simulink model "sampleModel2084"  (R2023a)
settings: Solver=VariableStepAuto  StartTime=0.0  StopTime=10.0  RelTol=1e-3
libraries: hdlsllib x5, simulink x3
settings Model: Creator=user1  LastModifiedBy=user1

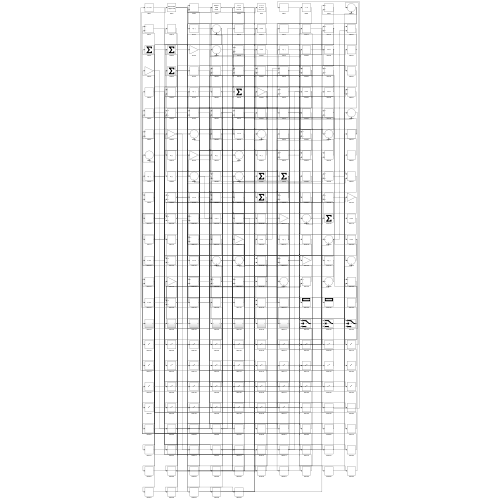
[thumbnail: Simulink's stored preview of the top-level diagram]
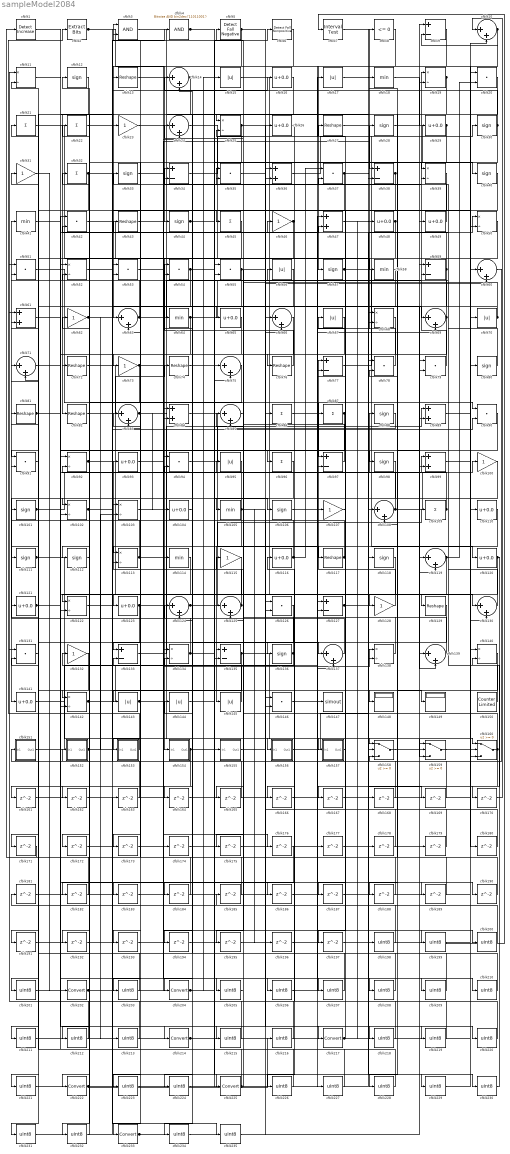
== system sampleModel2084 ==
  cfblk1 : simulink/Logic and Bit Operations/Detect Increase  vinit=0.0  OutDataTypeStr=boolean
      settings: LibrarySourceBlock=|
      | hdlsllib/Logic and Bit
      | Operations/Detect
      | Increase
  cfblk{10,14,24,60,63,66,69,71,75,83,85,108,119,124..125,130,137,139} (18 alike) : Sum  Inputs=|++
  cfblk{23,31,46,62,73,100,107,115,128,132} (10 alike) : Gain
  cfblk{12,28,30,33,40,44,57,80,88,98,101,106,111..112,118,136} (16 alike) : Signum
  cfblk{11,19,25,39,50,52,68,92,102..103,113,122,134,138,140,142} (16 alike) : Product  Inputs=*/  RndMeth=Zero  SaturateOnIntegerOverflow=on
  cfblk{16,26,29,48..49,65,93,104,110,116,120..121,123,141} (14 alike) : Bias  Bias=0.0  SaturateOnIntegerOverflow=off
  cfblk{18,41,58,64,105,114} (6 alike) : MinMax
  cfblk{21..22,32,45,86..87,96,109} (8 alike) : Sum  Inputs=+
  cfblk{13,27,43,72,74,76,81..82,117,129} (10 alike) : Reshape
  cfblk{20,35,37,42,51,53..55,78..79,90..91,94,126,131,146} (16 alike) : DotProduct  OutDataTypeStr=Inherit: Inherit via internal rule
  cfblk{9,34,38,59,77,97,127,133,135} (9 alike) : Sum  Inputs=+-
  cfblk{15,17,56,67,70,95,143..145} (9 alike) : Abs  SaturateOnIntegerOverflow=off
  cfblk147 : ToWorkspace  VariableName=simout  SaveFormat=Timeseries  SampleTime=-1
  cfblk148 : Display
  cfblk149 : Display
  cfblk150 : hdlsllib/Sources/Counter Limited  uplimit=7  tsamp=-1
  cfblk151 : Subsystem
      settings: LibrarySourceBlock=|
      | hdlsllib/Ports &
      | Subsystems/Subsystem
  cfblk152 : Subsystem
      settings: LibrarySourceBlock=|
      | hdlsllib/Ports &
      | Subsystems/Subsystem
  cfblk153 : Subsystem
      settings: LibrarySourceBlock=|
      | hdlsllib/Ports &
      | Subsystems/Subsystem
  cfblk154 : Subsystem
      settings: LibrarySourceBlock=|
      | hdlsllib/Ports &
      | Subsystems/Subsystem
  cfblk155 : Subsystem
      settings: LibrarySourceBlock=|
      | hdlsllib/Ports &
      | Subsystems/Subsystem
  cfblk156 : Subsystem
      settings: LibrarySourceBlock=|
      | hdlsllib/Ports &
      | Subsystems/Subsystem
  cfblk157 : Subsystem
      settings: LibrarySourceBlock=|
      | hdlsllib/Ports &
      | Subsystems/Subsystem
  cfblk158 : Switch  SaturateOnIntegerOverflow=off  InputSameDT=off
  cfblk159 : Switch  SaturateOnIntegerOverflow=off  InputSameDT=off
  cfblk160 : Switch  SaturateOnIntegerOverflow=off  InputSameDT=off
  cfblk{161..197} (37 alike) : Delay  SampleTime=1
  cfblk{198..201,203,205..213,215..216,218..221,223..224,226..232,234..235} (31 alike) : DataTypeConversion  OutDataTypeStr=uint8  SaturateOnIntegerOverflow=off  RndMeth=Floor
  cfblk2 : simulink/Logic and Bit Operations/Extract Bits  bitsToExtract=Upper half  numBits=8  bitIdxRange=[0 7]  outScalingMode=Preserve fixed-point scaling
      settings: LibrarySourceBlock=|
      | hdlsllib/Logic and Bit
      | Operations/Extract Bits
  cfblk{202,204,214,217,222,225,233} (7 alike) : DataTypeConversion  SaturateOnIntegerOverflow=off  RndMeth=Floor
  cfblk3 : Logic  AllPortsSameDT=off  OutDataTypeStr=boolean
  cfblk{36,47,61,84,89,99} (6 alike) : Sum
  cfblk4 : simulink/Logic and Bit Operations/Bitwise Operator  logicop=AND  UseBitMask=on  BitMask=bin2dec('11011001')  BitMaskRealWorld=Stored Integer
      settings: LibrarySourceBlock=|
      | hdlsllib/Logic and Bit
      | Operations/Bitwise
      | Operator
  cfblk5 : hdlsllib/Logic and Bit Operations/Detect Fall Negative  vinit=0  OutDataTypeStr=boolean
  cfblk6 : hdlsllib/Logic and Bit Operations/Detect Fall Nonpositive  vinit=0  OutDataTypeStr=boolean
  cfblk7 : hdlsllib/Logic and Bit Operations/Interval Test  IntervalClosedRight=on  uplimit=0.5  IntervalClosedLeft=on  lowlimit=-0.5  OutDataTypeStr=boolean
  cfblk8 : hdlsllib/Logic and Bit Operations/Compare To Zero  relop=<=  OutDataTypeStr=boolean
  wires:
  cfblk20/1 -> cfblk82/1
  cfblk78/1 -> cfblk8/1
  cfblk100/1 -> cfblk141/1
  cfblk153/1(Out1) -> cfblk2/1
  cfblk8/1 -> cfblk63/1
  cfblk60/1 -> cfblk151/1(In1)
  cfblk117/1 -> cfblk41/1, cfblk64/1
  cfblk130/1 -> cfblk33/1
  cfblk5/1 -> cfblk13/1, cfblk38/2, cfblk98/1
  cfblk29/1 -> cfblk153/1(In1), cfblk76/1
  cfblk115/1 -> cfblk204/1
  cfblk79/1 -> cfblk19/1
  cfblk81/1 -> cfblk128/1, cfblk96/1
  cfblk13/1 -> cfblk156/1(In1)
  cfblk128/1 -> cfblk77/1
  cfblk25/1 -> cfblk130/1, cfblk122/1
  cfblk6/1 -> cfblk44/1
  cfblk72/1 -> cfblk129/1
  cfblk108/1 -> cfblk100/1, cfblk32/1
  cfblk73/1 -> cfblk28/1, cfblk90/1, cfblk172/1
  cfblk158/1 -> cfblk119/1
  cfblk77/1 -> cfblk30/1
  cfblk69/1 -> cfblk54/2, cfblk226/1
  cfblk9/1 -> cfblk57/1
  cfblk107/1 -> cfblk27/1
  cfblk21/1 -> cfblk154/1(In1)
  cfblk83/1 -> cfblk148/1, cfblk104/1
  cfblk52/1 -> cfblk225/1
  cfblk121/1 -> cfblk81/1, cfblk215/1
  cfblk56/1 -> cfblk123/1
  cfblk136/1 -> cfblk24/1, cfblk134/2
  cfblk127/1 -> cfblk50/1, cfblk159/3
  cfblk19/1 -> cfblk25/1, cfblk108/2
  cfblk64/1 -> cfblk56/1, cfblk142/2
  cfblk59/1 -> cfblk84/1, cfblk22/1
  cfblk84/1 -> cfblk117/1
  cfblk57/1 -> cfblk120/1, cfblk139/2
  cfblk24/1 -> cfblk147/1
  cfblk37/1 -> cfblk122/2, cfblk169/1
  cfblk68/1 -> cfblk133/1
  cfblk51/1 -> cfblk97/1
  cfblk109/1 -> cfblk62/1, cfblk18/1
  cfblk104/1 -> cfblk34/1
  cfblk36/1 -> cfblk9/1
  cfblk54/1 -> cfblk91/1, cfblk106/1, cfblk186/1
  cfblk10/1 -> cfblk127/2, cfblk160/2, cfblk9/2
  cfblk61/1 -> cfblk217/1
  cfblk34/1 -> cfblk17/1
  cfblk113/1 -> cfblk93/1, cfblk208/1
  cfblk14/1 -> cfblk72/1, cfblk221/1
  cfblk135/1 -> cfblk158/1, cfblk142/1
  cfblk15/1 -> cfblk107/1
  cfblk92/1 -> cfblk137/1, cfblk90/2
  cfblk82/1 -> cfblk74/1
  cfblk133/1 -> cfblk89/1
  cfblk1/1 -> cfblk23/1
  cfblk125/1 -> cfblk103/1, cfblk113/2
  cfblk105/1 -> cfblk102/1, cfblk113/1, cfblk196/1, cfblk207/1
  cfblk139/1 -> cfblk5/1
  cfblk156/1(Out1) -> cfblk78/1
  cfblk154/1(Out1) -> cfblk15/1, cfblk171/1
  cfblk48/1 -> cfblk94/1, cfblk101/1
  cfblk138/1 -> cfblk85/1
  cfblk120/1 -> cfblk143/1, cfblk170/1
  cfblk80/1 -> cfblk51/2
  cfblk2/1 -> cfblk24/2, cfblk99/2, cfblk50/2
  cfblk103/1 -> cfblk88/1
  cfblk97/1 -> cfblk3/1
  cfblk134/1 -> cfblk91/2, cfblk14/2, cfblk230/1
  cfblk76/1 -> cfblk54/1
  cfblk146/1 -> cfblk138/1
  cfblk30/1 -> cfblk39/1, cfblk14/1
  cfblk111/1 -> cfblk160/1, cfblk43/1
  cfblk110/1 -> cfblk145/1
  cfblk75/1 -> cfblk222/1
  cfblk43/1 -> cfblk149/1
  cfblk4/1 -> cfblk40/1, cfblk58/1
  cfblk32/1 -> cfblk16/1, cfblk146/2, cfblk111/1
  cfblk66/1 -> cfblk233/1
  cfblk28/1 -> cfblk110/1
  cfblk159/1 -> cfblk80/1
  cfblk31/1 -> cfblk202/1
  cfblk3/1 -> cfblk118/1
  cfblk143/1 -> cfblk138/2, cfblk39/2
  cfblk94/1 -> cfblk36/2
  cfblk119/1 -> cfblk20/2, cfblk125/2, cfblk232/1
  cfblk50/1 -> cfblk112/1
  cfblk27/1 -> cfblk38/1
  cfblk152/1(Out1) -> cfblk4/1, cfblk103/2, cfblk182/1
  cfblk102/1 -> cfblk12/1, cfblk205/1
  cfblk55/1 -> cfblk60/2, cfblk105/1, cfblk164/1
  cfblk42/1 -> cfblk108/1
  cfblk116/1 -> cfblk83/1, cfblk37/1
  cfblk89/1 -> cfblk10/2
  cfblk137/1 -> cfblk124/1
  cfblk87/1 -> cfblk102/2, cfblk173/1
  cfblk11/1 -> cfblk214/1
  cfblk155/1(Out1) -> cfblk126/1
  cfblk88/1 -> cfblk85/2
  cfblk95/1 -> cfblk124/2
  cfblk141/1 -> cfblk68/2
  cfblk38/1 -> cfblk34/2, cfblk45/1
  cfblk124/1 -> cfblk109/1, cfblk157/1(In1)
  cfblk142/1 -> cfblk69/2, cfblk192/1
  cfblk70/1 -> cfblk35/1, cfblk65/1
  cfblk33/1 -> cfblk134/1
  cfblk145/1 -> cfblk92/2
  cfblk160/1 -> cfblk95/1, cfblk197/1
  cfblk63/1 -> cfblk21/1, cfblk59/2
  cfblk151/1(Out1) -> cfblk53/2
  cfblk45/1 -> cfblk73/1
  cfblk46/1 -> cfblk136/1, cfblk83/2
  cfblk150/1 -> cfblk46/1
  cfblk123/1 -> cfblk190/1, cfblk191/1
  cfblk35/1 -> cfblk87/1
  cfblk118/1 -> cfblk135/1
  cfblk122/1 -> cfblk47/2
  cfblk18/1 -> cfblk29/1
  cfblk22/1 -> cfblk69/1
  cfblk101/1 -> cfblk49/1, cfblk99/1
  cfblk62/1 -> cfblk213/1, cfblk235/1
  cfblk49/1 -> cfblk35/2
  cfblk74/1 -> cfblk6/1
  cfblk44/1 -> cfblk114/1, cfblk160/3
  cfblk91/1 -> cfblk161/1
  cfblk161/1 -> cfblk130/2
  cfblk112/1 -> cfblk162/1
  cfblk162/1 -> cfblk89/2
  cfblk163/1 -> cfblk42/2
  cfblk164/1 -> cfblk19/2
  cfblk85/1 -> cfblk165/1
  cfblk165/1 -> cfblk53/1
  cfblk26/1 -> cfblk166/1
  cfblk166/1 -> cfblk127/1
  cfblk39/1 -> cfblk167/1
  cfblk167/1 -> cfblk159/2
  cfblk17/1 -> cfblk168/1
  cfblk168/1 -> cfblk68/1
  cfblk169/1 -> cfblk159/1
  cfblk170/1 -> cfblk10/1
  cfblk171/1 -> cfblk1/1
  cfblk172/1 -> cfblk139/1
  cfblk173/1 -> cfblk3/2
  cfblk126/1 -> cfblk175/1
  cfblk93/1 -> cfblk176/1
  cfblk177/1 -> cfblk79/2
  cfblk178/1 -> cfblk37/2
  cfblk179/1 -> cfblk78/2
  cfblk99/1 -> cfblk180/1
  cfblk180/1 -> cfblk36/1
  cfblk181/1 -> cfblk119/2
  cfblk182/1 -> cfblk92/1
  cfblk40/1 -> cfblk183/1
  cfblk183/1 -> cfblk20/1
  cfblk58/1 -> cfblk184/1
  cfblk184/1 -> cfblk133/2
  cfblk185/1 -> cfblk94/2
  cfblk186/1 -> cfblk137/2
  cfblk157/1(Out1) -> cfblk187/1
  cfblk187/1 -> cfblk77/2
  cfblk90/1 -> cfblk188/1
  cfblk188/1 -> cfblk63/2
  cfblk41/1 -> cfblk189/1
  cfblk189/1 -> cfblk51/1
  cfblk190/1 -> cfblk158/3
  cfblk191/1 -> cfblk135/2
  cfblk192/1 -> cfblk60/1
  cfblk67/1 -> cfblk193/1
  cfblk193/1 -> cfblk47/1
  cfblk129/1 -> cfblk194/1
  cfblk194/1 -> cfblk158/2
  cfblk96/1 -> cfblk195/1
  cfblk195/1 -> cfblk25/2
  cfblk196/1 -> cfblk97/2
  cfblk7/1 -> cfblk198/1
  cfblk198/1 -> cfblk121/1
  cfblk53/1 -> cfblk199/1
  cfblk199/1 -> cfblk7/1
  cfblk174/1 -> cfblk200/1
  cfblk200/1 -> cfblk55/1
  cfblk12/1 -> cfblk201/1
  cfblk201/1 -> cfblk174/1
  cfblk202/1 -> cfblk84/2, cfblk55/2
  cfblk114/1 -> cfblk203/1
  cfblk203/1 -> cfblk31/1
  cfblk204/1 -> cfblk125/1, cfblk155/1(In1)
  cfblk205/1 -> cfblk115/1
  cfblk71/1 -> cfblk206/1
  cfblk206/1 -> cfblk177/1
  cfblk207/1 -> cfblk71/1
  cfblk208/1 -> cfblk71/2
  cfblk144/1 -> cfblk209/1
  cfblk209/1 -> cfblk79/1
  cfblk23/1 -> cfblk210/1
  cfblk210/1 -> cfblk144/1
  cfblk131/1 -> cfblk211/1
  cfblk211/1 -> cfblk70/1
  cfblk176/1 -> cfblk212/1
  cfblk212/1 -> cfblk131/1
  cfblk213/1 -> cfblk131/2
  cfblk214/1 -> cfblk26/1, cfblk146/1
  cfblk215/1 -> cfblk11/1
  cfblk216/1 -> cfblk11/2
  cfblk217/1 -> cfblk67/1, cfblk59/1, cfblk48/1
  cfblk175/1 -> cfblk218/1
  cfblk218/1 -> cfblk61/1
  cfblk47/1 -> cfblk219/1
  cfblk219/1 -> cfblk61/2
  cfblk86/1 -> cfblk220/1
  cfblk220/1 -> cfblk116/1
  cfblk221/1 -> cfblk86/1
  cfblk222/1 -> cfblk216/1, cfblk178/1
  cfblk65/1 -> cfblk223/1
  cfblk223/1 -> cfblk75/1
  cfblk16/1 -> cfblk224/1
  cfblk224/1 -> cfblk75/2
  cfblk225/1 -> cfblk185/1, cfblk181/1, cfblk152/1(In1)
  cfblk226/1 -> cfblk52/1
  cfblk106/1 -> cfblk227/1
  cfblk227/1 -> cfblk52/2
  cfblk140/1 -> cfblk228/1
  cfblk228/1 -> cfblk42/1
  cfblk197/1 -> cfblk229/1
  cfblk229/1 -> cfblk140/1
  cfblk230/1 -> cfblk140/2
  cfblk132/1 -> cfblk231/1
  cfblk231/1 -> cfblk163/1
  cfblk232/1 -> cfblk132/1
  cfblk233/1 -> cfblk179/1, cfblk126/2
  cfblk98/1 -> cfblk234/1
  cfblk234/1 -> cfblk66/1
  cfblk235/1 -> cfblk66/2

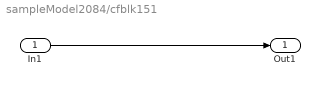
== system sampleModel2084/cfblk151 ==
  In1 : Inport
  Out1 : Outport
  wires:
  In1/1 -> Out1/1

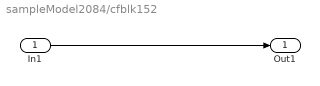
== system sampleModel2084/cfblk152 ==
  In1 : Inport
  Out1 : Outport
  wires:
  In1/1 -> Out1/1

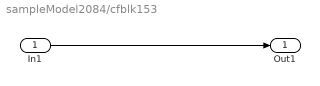
== system sampleModel2084/cfblk153 ==
  In1 : Inport
  Out1 : Outport
  wires:
  In1/1 -> Out1/1

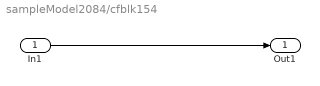
== system sampleModel2084/cfblk154 ==
  In1 : Inport
  Out1 : Outport
  wires:
  In1/1 -> Out1/1

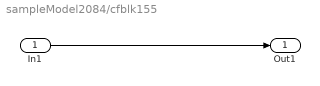
== system sampleModel2084/cfblk155 ==
  In1 : Inport
  Out1 : Outport
  wires:
  In1/1 -> Out1/1

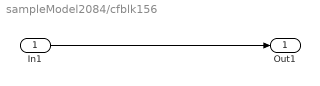
== system sampleModel2084/cfblk156 ==
  In1 : Inport
  Out1 : Outport
  wires:
  In1/1 -> Out1/1

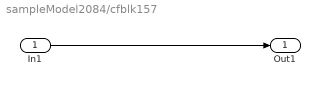
== system sampleModel2084/cfblk157 ==
  In1 : Inport
  Out1 : Outport
  wires:
  In1/1 -> Out1/1
